simulink model "balancesim"  (R2012b)
settings: Solver=ode3  StartTime=0.0  StopTime=inf  FixedStep=0.001  RelTol=1e-3
undefined symbols (not defined in the file or in its folder): HIL, qc_get_step_size
libraries: quarc_library x7
settings Model: SimulationMode=external  ExtModeTrigDuration=15000  Creator=runkunwang  LastModifiedBy=runkunwang
settings SolverCC: PositivePriorityOrder=on
settings RTWCC: SystemTargetFile=quarc_win64.tlc  TemplateMakefile=quarc_default_tmf  Description=QUARC Win64 Target  ProcessScript=quarc_win64_make_rtw_hook
settings STFCustomTargetCC: TargetPreCompLibLocation=C:\PROGRA~3\QUARC\lib\2012b\win64\release  CodeReplacementLibrary=ANSI_C  GeneratePreprocessorConditionals=Disable all  CombineOutputUpdateFcns=on  GRTInterface=off  SystemTargetFile=quarc_win64.tlc
settings GRTTargetCC: TargetPreCompLibLocation=C:\PROGRA~3\QUARC\lib\2012b\win64\release  ParMdlRefBuildCompliant=off  CompOptLevelCompliant=off  ConcurrentExecutionCompliant=off  MatFileLogging=off  ExtMode=on  ExtModeMexFile=quarc_comm

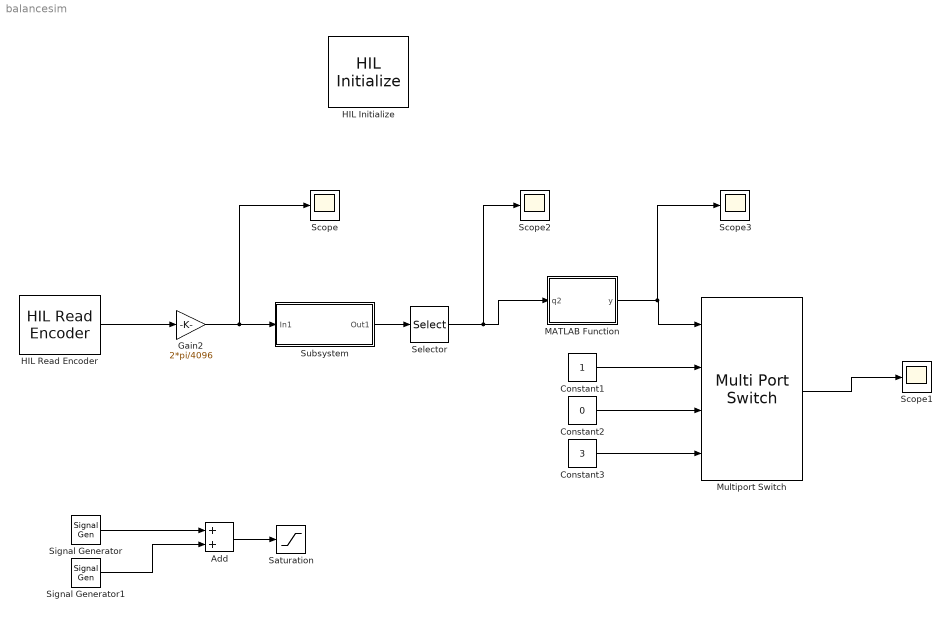
== system balancesim ==
  Add : Sum
  Constant1 : Constant
  Constant2 : Constant  Value=0
  Constant3 : Constant  Value=3
  Gain2 : Gain  Gain=2*pi/4096  ParamMin=[-512]  ParamMax=[512]
  HIL Initialize : quarc_library/Data Acquisition/Generic/Configuration/HIL Initialize  Priority=-99  object_name=HIL-1  board_type=q2_usb  board_number=0  board_options=d0=digital;d1=digital;led=auto;update_rate=normal;decimation=1  exclusive=off  active=off  hardware_clocks=[0]  clock_modes=[]  initial_clock_frequencies=[]  set_clock_params_at_start=off  set_clock_params_at_switch_in=off  set_clock_frequencies_at_start=off  set_clock_frequencies_at_switch_in=off  analog_input_channels=[0:1]  analog_input_maximums=10  analog_input_minimums=-10  set_analog_input_params_at_start=on  set_analog_input_params_at_switch_in=off  analog_output_channels=[0:1]  analog_output_maximums=10  analog_output_minimums=-10  initial_analog_outputs=[0]  final_analog_outputs=[0]  watchdog_analog_outputs=0  set_analog_output_params_at_start=on  set_analog_output_params_at_switch_in=off  set_analog_outputs_at_start=on  set_analog_outputs_at_switch_in=off  set_analog_outputs_at_terminate=on  set_analog_outputs_at_switch_out=off  set_analog_outputs_on_watchdog=off  digital_input_channels=[]  digital_output_channels=[]  digital_output_configuration=[]  initial_digital_outputs=[1]  final_digital_outputs=[1]  watchdog_digital_outputs=[1]  set_digital_output_params_at_start=off  set_digital_output_params_at_switch_in=off  set_digital_outputs_at_start=on  set_digital_outputs_at_switch_in=off  set_digital_outputs_at_terminate=on  set_digital_outputs_at_switch_out=off  set_digital_outputs_on_watchdog=off  encoder_channels=[0:1]  quadrature=[4]  encoder_filter_frequency=[]  initial_encoder_counts=[0]  set_encoder_params_at_start=on  set_encoder_params_at_switch_in=off  set_encoder_counts_at_start=on  set_encoder_counts_at_switch_in=off  pwm_channels=[]  pwm_modes=[0]  pwm_frequency=1/0.020  pwm_configuration=[]  pwm_alignment=[]  pwm_polarity=[]  pwm_leading_deadband=[]  pwm_trailing_deadband=[]  initial_pwm_outputs=[0]  final_pwm_outputs=[0]  watchdog_pwm_outputs=[0]  set_pwm_params_at_start=on  set_pwm_params_at_switch_in=off  set_pwm_outputs_at_start=on  set_pwm_outputs_at_switch_in=off  set_pwm_outputs_at_terminate=on  set_pwm_outputs_at_switch_out=off  set_pwm_outputs_on_watchdog=off  other_output_channels=[]  initial_other_outputs=[]  final_other_outputs=[]  watchdog_other_outputs=[]  set_other_outputs_at_start=off  set_other_outputs_at_switch_in=off  set_other_outputs_at_terminate=off  set_other_outputs_at_switch_out=off  set_other_outputs_on_watchdog=off
  HIL Read Encoder : quarc_library/Data Acquisition/Generic/Immediate I//O/HIL Read Encoder  object_name=HIL-1  channels=1  sample_time=qc_get_step_size  active=on  vector_output=off  data_type_mode=Inherit via back propagation  data_type=double
  MATLAB Function : MATLAB Function  TreatAsAtomicUnit=on
  Multiport Switch : MultiPortSwitch
  Saturation : Saturate  UpperLimit=10  LowerLimit=-10
  Scope{,1..3} (4 alike) : Scope
      Scope2 settings: YMin=-13.5  YMax=-3  SaveName=ScopeData2  MaxDataPoints=10000
      Scope3 settings: SaveName=ScopeData3  MaxDataPoints=10000
  Selector : Selector  InputPortWidth=5  IndexOptions=Index vector (dialog)  Indices=[4]  OutputSizes=1
  Signal Generator : SignalGenerator  Frequency=5
  Signal Generator1 : SignalGenerator  Amplitude=10  Frequency=sqrt(2)
  Subsystem : Subsystem
  wires:
  MATLAB Function/1(y) -> Scope3/1, Multiport Switch/1
  Multiport Switch/1 -> Scope1/1
  Constant3/1 -> Multiport Switch/4
  Constant2/1 -> Multiport Switch/3
  Constant1/1 -> Multiport Switch/2
  Selector/1 -> Scope2/1, MATLAB Function/1(q2)
  Subsystem/1(Out1) -> Selector/1
  Add/1 -> Saturation/1
  Signal Generator/1 -> Add/1
  Signal Generator1/1 -> Add/2
  Gain2/1 -> Scope/1, Subsystem/1(In1)
  HIL Read Encoder/1 -> Gain2/1

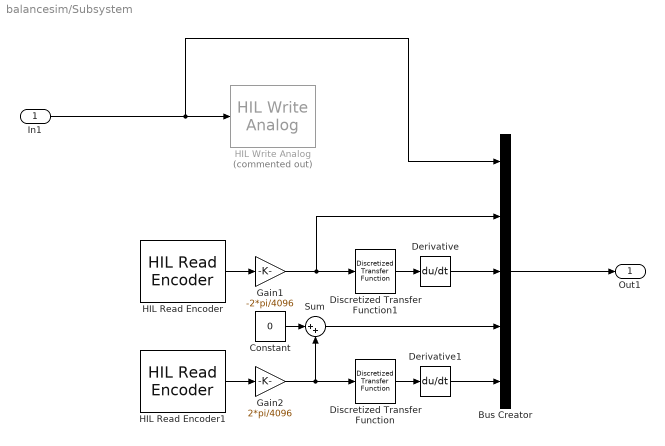
== system balancesim/Subsystem ==
  In1 : Inport
  Bus Creator : BusCreator  Inputs=5
  Constant : Constant  Value=0
  Derivative : Derivative
  Derivative1 : Derivative
  Discretized Transfer Function : quarc_library/Discrete/Discretized Transfer Function  num=100  den=[1 100]  method=tustin  Ts=qc_get_step_size
  Discretized Transfer Function1 : quarc_library/Discrete/Discretized Transfer Function  num=100  den=[1 100]  method=tustin  Ts=qc_get_step_size
  Gain1 : Gain  Gain=-2*pi/4096  ParamMin=[-512]  ParamMax=[512]
  Gain2 : Gain  Gain=2*pi/4096  ParamMin=[-512]  ParamMax=[512]
  HIL Read Encoder : quarc_library/Data Acquisition/Generic/Immediate I//O/HIL Read Encoder  object_name=HIL-1  channels=0  sample_time=qc_get_step_size  active=on  vector_output=off  data_type_mode=Inherit via back propagation  data_type=double
  HIL Read Encoder1 : quarc_library/Data Acquisition/Generic/Immediate I//O/HIL Read Encoder  object_name=HIL-1  channels=1  sample_time=qc_get_step_size  active=on  vector_output=off  data_type_mode=Inherit via back propagation  data_type=double
  HIL Write Analog : quarc_library/Data Acquisition/Generic/Immediate I//O/HIL Write Analog  Commented=on  object_name=HIL-1  channels=0  sample_time=-1  active=off  vector_input=off
  Sum : Sum  Inputs=|++
  Out1 : Outport
  wires:
  HIL Read Encoder/1 -> Gain1/1
  HIL Read Encoder1/1 -> Gain2/1
  Gain1/1 -> Bus Creator/2, Discretized Transfer Function1/1
  Gain2/1 -> Discretized Transfer Function/1, Sum/2
  Discretized Transfer Function1/1 -> Derivative/1
  Discretized Transfer Function/1 -> Derivative1/1
  Derivative/1 -> Bus Creator/3
  Derivative1/1 -> Bus Creator/5
  Constant/1 -> Sum/1
  Sum/1 -> Bus Creator/4
  In1/1 -> Bus Creator/1, HIL Write Analog/1
  Bus Creator/1 -> Out1/1

== matlab function balancesim/MATLAB Function ==
  data: q2 input; y output
function y = fcn(q2)

y = 2;
if q2 < 0
    q2 = -q2;
end
if q2 >= 2*pi 
    q2 = mod(q2, 2*pi);
end
%Zone 3
if q2 >= (8*pi)/9 || q2 <= (10*pi)/9
        y = 3;
end
%Zone 2        
if (q2 > pi/18 && q2 < (8*pi)/9) || (q2 > (10*pi)/9 && q2 < (35*pi)/18)
        y = 2;
end
%Zone 1        
if q2 <= (pi)/18 || q2 >= mod((35*pi)/18,2*pi)
        y = 1;
end
